simulink model "Impedance_Controller_Week5"  (R2015b)
settings: Solver=ode23t  StartTime=0.0  StopTime=20  MaxStep=1.2  RelTol=1e-5
values from neighbouring files (symbols this model uses):
  B = 0    [ME_495_Position_Control_1.m]    (also in PI_Controller_Week5.m; PI_controller_win1_simulink.m)
  B_desired = testcase(3,i)    [ME_495_Position_Control_1.m]    (also in PI_Controller_Week5.m; PI_controller_win1_simulink.m; TEST.m)
  c = 2*pi*r    (= 0.0552920307032)    [ME_495_Position_Control_1.m]    (also in PI_Controller_Week5.m; PI_controller_win1_simulink.m)
  Fss = testcase(4,i)    [ME_495_Position_Control_1.m]    (also in PI_Controller_Week5.m; PI_controller_win1_simulink.m; TEST.m = 20)
  impulse_duration = input('Duration of the impulse = ')    [ME_495_Position_Control_1.m]    (also in PI_Controller_Week5.m; PI_controller_win1_simulink.m)
  input_mode = input('input mode = ')    [ME_495_Position_Control_1.m]    (also in PI_Controller_Week5.m; PI_controller_win1_simulink.m)
  J = .001    (= 0.001)    [ME_495_Position_Control_1.m]    (also in PI_Controller_Week5.m; PI_controller_win1_simulink.m)
  K_desired = testcase(2,i)    [ME_495_Position_Control_1.m]    (also in PI_Controller_Week5.m; PI_controller_win1_simulink.m; TEST.m)
  Ka = .79    (= 0.79)    [ME_495_Position_Control_1.m]    (also in PI_Controller_Week5.m; PI_controller_win1_simulink.m)
  Ki = wn^2*(r*(M+J*((N^2)/(r^2))))/Ka/Km/N    [PI_Controller_Week5.m]    (also in PI_controller_win1_simulink.m = -f*x*Kp)
  Km = .058    (= 0.058)    [ME_495_Position_Control_1.m]    (also in PI_Controller_Week5.m; PI_controller_win1_simulink.m = 0.11)
  Kp = (wn^2)*r*(M+J/((N*r)^2))/(Ka*Km*N)    [ME_495_Position_Control_1.m]    (also in PI_Controller_Week5.m = (2*zeta*wn*(r*(M+J*((N^2)/(r^2))))-B/r)/(Ka*Km*N); PI_controller_win1_simulink.m = (2*zeta*wn*(r*(M+J/(r^2)))-B/r)/(Ka*Km))
  M = 1    [ME_495_Position_Control_1.m]    (also in PI_Controller_Week5.m; PI_controller_win1_simulink.m; TEST.m)
  M_desired = testcase(1,i)    [ME_495_Position_Control_1.m]    (also in PI_Controller_Week5.m; PI_controller_win1_simulink.m; TEST.m)
  N = 5.9    [ME_495_Position_Control_1.m]    (also in PI_Controller_Week5.m)
  override_flag = 1    [ME_495_Position_Control_1.m]    (also in PI_Controller_Week5.m; PI_controller_win1_simulink.m)
  r = .0176/2    (= 0.0088)    [ME_495_Position_Control_1.m]    (also in PI_Controller_Week5.m; PI_controller_win1_simulink.m)
  Rmot = 3.91    [ME_495_Position_Control_1.m]    (also in PI_Controller_Week5.m = 4; PI_controller_win1_simulink.m = 4)
  target_speed = 5    [ME_495_Position_Control_1.m]    (also in PI_Controller_Week5.m; PI_controller_win1_simulink.m)
  vol_limit = 24    [PI_Controller_Week5.m]
libraries: simulink x3
settings Model: Creator=Jeff  LastModifiedBy=Jeff

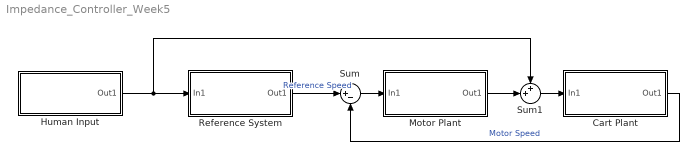
== system Impedance_Controller_Week5 ==
  Cart Plant : Subsystem
  Human Input : Subsystem
  Motor Plant : Subsystem
  Reference System : Subsystem
  Sum : Sum  Inputs=|+-
  Sum1 : Sum  Inputs=++|
  wires:
  Reference System/1(Out1) -> Sum/1  "Reference Speed"
  Cart Plant/1(Out1) -> Sum/2  "Motor Speed"
  Sum1/1 -> Cart Plant/1(In1)
  Sum/1 -> Motor Plant/1(In1)
  Human Input/1(Out1) -> Reference System/1(In1), Sum1/1
  Motor Plant/1(Out1) -> Sum1/2

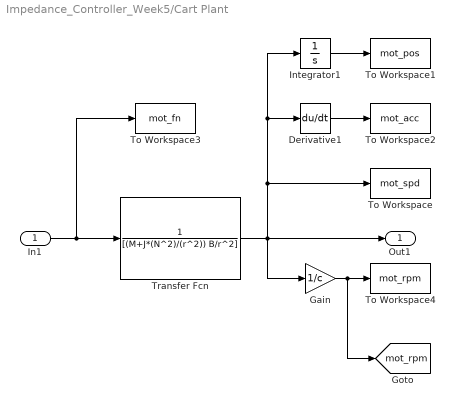
== system Impedance_Controller_Week5/Cart Plant ==
  In1 : Inport
  Derivative1 : Derivative
  Gain : Gain  Gain=1/c
  Integrator1 : Integrator
  To Workspace : ToWorkspace  VariableName=mot_spd  SaveFormat=Timeseries  SampleTime=-1
  To Workspace1 : ToWorkspace  VariableName=mot_pos  SaveFormat=Timeseries  SampleTime=-1
  To Workspace2 : ToWorkspace  VariableName=mot_acc  SaveFormat=Timeseries  SampleTime=-1
  To Workspace3 : ToWorkspace  VariableName=mot_fn  SaveFormat=Timeseries  SampleTime=-1
  To Workspace4 : ToWorkspace  VariableName=mot_rpm  SaveFormat=Timeseries  SampleTime=-1
  Transfer Fcn : TransferFcn  Denominator=[(M+J*(N^2)/(r^2)) B/r^2]
  Out1 : Outport
  tag scope: mot_rpm=global
  wires:
  Integrator1/1 -> To Workspace1/1
  Derivative1/1 -> To Workspace2/1
  In1/1 -> To Workspace3/1, Transfer Fcn/1
  Gain/1 -> [mot_rpm], To Workspace4/1
  Transfer Fcn/1 -> Gain/1, Out1/1, Integrator1/1, Derivative1/1, To Workspace/1

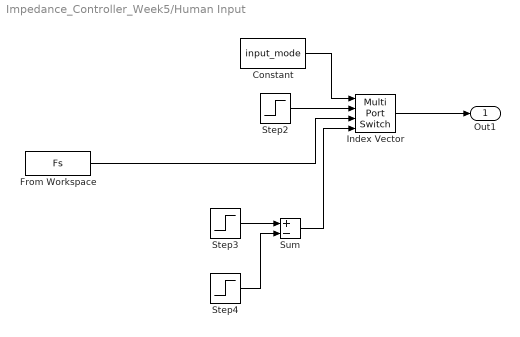
== system Impedance_Controller_Week5/Human Input ==
  Constant : Constant  Value=input_mode
  From Workspace : FromWorkspace  VariableName=Fs  SampleTime=0
  Index Vector : MultiPortSwitch  DataPortOrder=Zero-based contiguous  zeroidx=on
  Step2 : Step  Time=0  After=Fss  SampleTime=0
  Step3 : Step  Time=0  After=Fss  SampleTime=0
  Step4 : Step  Time=impulse_duration  After=Fss  SampleTime=0
  Sum : Sum  Inputs=+-
  Out1 : Outport
  wires:
  From Workspace/1 -> Index Vector/3
  Step2/1 -> Index Vector/2
  Index Vector/1 -> Out1/1
  Constant/1 -> Index Vector/1
  Sum/1 -> Index Vector/4
  Step3/1 -> Sum/1
  Step4/1 -> Sum/2

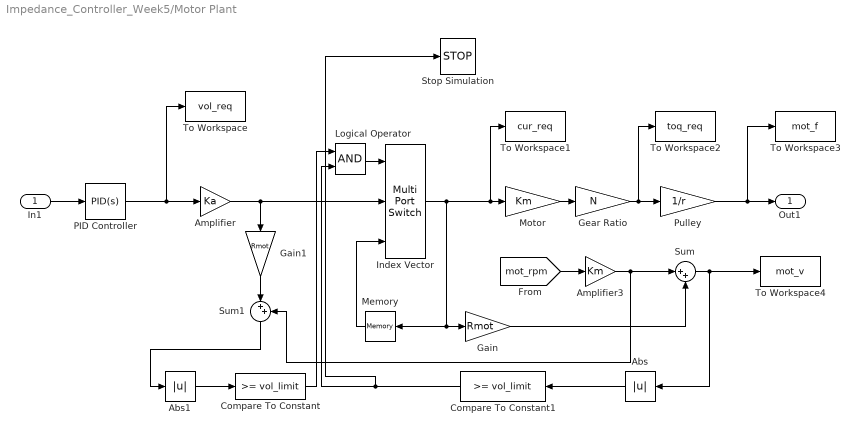
== system Impedance_Controller_Week5/Motor Plant ==
  In1 : Inport
  Abs : Abs
  Abs1 : Abs
  Amplifier : Gain  Gain=Ka
  Amplifier3 : Gain  Gain=Km
  Compare To Constant : simulink/Logic and Bit Operations/Compare To Constant  relop=>=  const=vol_limit  OutDataTypeStr=boolean
  Compare To Constant1 : simulink/Logic and Bit Operations/Compare To Constant  relop=>=  const=vol_limit  OutDataTypeStr=boolean
  Gain : Gain  Gain=Rmot
  Gain1 : Gain  Gain=Rmot
  Gear Ratio : Gain  Gain=N
  Index Vector : MultiPortSwitch  DataPortOrder=Zero-based contiguous  Inputs=2  zeroidx=on
  Logical Operator : Logic  AllPortsSameDT=off  OutDataTypeStr=boolean
  Memory : Memory
  Motor : Gain  Gain=Km
  PID Controller : simulink/Continuous/PID Controller  Controller=PID  TimeDomain=Continuous-time  SampleTime=-1  IntegratorMethod=Forward Euler  FilterMethod=Forward Euler  Form=Parallel  UseFilter=on  ControllerParametersSource=internal  P=Kp  I=Ki  D=0  N=100  InitialConditionSource=internal  InitialConditionForIntegrator=0  InitialConditionForFilter=0  ExternalReset=none  LimitOutput=off  UpperSaturationLimit=inf  LowerSaturationLimit=-inf  LinearizeAsGain=on  AntiWindupMode=none  Kb=1  TrackingMode=off  Kt=1  PParamMin=[]  PParamMax=[]  IParamMin=[]  IParamMax=[]  DParamMin=[]  DParamMax=[]  NParamMin=[]  NParamMax=[]  KbParamMin=[]  KbParamMax=[]  KtParamMin=[]  KtParamMax=[]  POutMin=[]  POutMax=[]  IOutMin=[]  IOutMax=[]  DOutMin=[]  DOutMax=[]  NOutMin=[]  NOutMax=[]  KbOutMin=[]  KbOutMax=[]  KtOutMin=[]  KtOutMax=[]  IntegratorOutMin=[]  IntegratorOutMax=[]  FilterOutMin=[]  FilterOutMax=[]  SumOutMin=[]  SumOutMax=[]  SumI1OutMin=[]  SumI1OutMax=[]  SumI2OutMin=[]  SumI2OutMax=[]  SumI3OutMin=[]  SumI3OutMax=[]  SumDOutMin=[]  SumDOutMax=[]  SaturationOutMin=[]  SaturationOutMax=[]  IntegratorContinuousStateAttributes=''  IntegratorStateMustResolveToSignalObject=off  IntegratorRTWStateStorageClass=Auto  FilterContinuousStateAttributes=''  FilterStateMustResolveToSignalObject=off  FilterRTWStateStorageClass=Auto  DifferentiatorICPrevScaledInput=0  DifferentiatorOutMin=[]  DifferentiatorOutMax=[]
  Pulley : Gain  Gain=1/r
  Stop Simulation : Stop
  Sum : Sum  Inputs=|++
  Sum1 : Sum  Inputs=|++
  To Workspace : ToWorkspace  VariableName=vol_req  SaveFormat=Timeseries  SampleTime=-1
  To Workspace1 : ToWorkspace  VariableName=cur_req  SaveFormat=Timeseries  SampleTime=-1
  To Workspace2 : ToWorkspace  VariableName=toq_req  SaveFormat=Timeseries  SampleTime=-1
  To Workspace3 : ToWorkspace  VariableName=mot_f  SaveFormat=Timeseries  SampleTime=-1
  To Workspace4 : ToWorkspace  VariableName=mot_v  SaveFormat=Timeseries  SampleTime=-1
  Out1 : Outport
  wires:
  In1/1 -> PID Controller/1
  Index Vector/1 -> Memory/1, Gain/1, To Workspace1/1, Motor/1
  Pulley/1 -> To Workspace3/1, Out1/1
  Gain/1 -> Sum/2
  Amplifier3/1 -> Sum/1, Sum1/2
  Sum/1 -> Abs/1, To Workspace4/1
  [mot_rpm] -> Amplifier3/1
  Motor/1 -> Gear Ratio/1
  Gear Ratio/1 -> To Workspace2/1, Pulley/1
  PID Controller/1 -> To Workspace/1, Amplifier/1
  Amplifier/1 -> Gain1/1, Index Vector/2
  Memory/1 -> Index Vector/3
  Gain1/1 -> Sum1/1
  Sum1/1 -> Abs1/1
  Compare To Constant/1 -> Logical Operator/1
  Logical Operator/1 -> Index Vector/1
  Abs/1 -> Compare To Constant1/1
  Abs1/1 -> Compare To Constant/1
  Compare To Constant1/1 -> Stop Simulation/1, Logical Operator/2

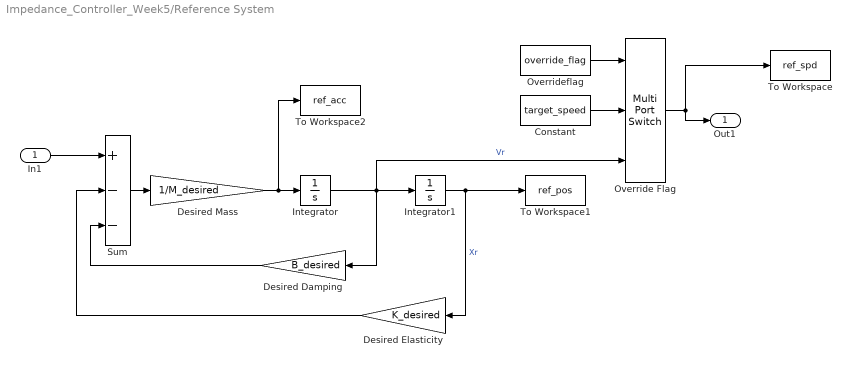
== system Impedance_Controller_Week5/Reference System ==
  In1 : Inport
  Constant : Constant  Value=target_speed
  Desired Damping : Gain  Gain=B_desired
  Desired Elasticity : Gain  Gain=K_desired
  Desired Mass : Gain  Gain=1/M_desired
  Integrator : Integrator
  Integrator1 : Integrator
  Override Flag : MultiPortSwitch  DataPortOrder=Zero-based contiguous  Inputs=2  zeroidx=on
  Overrideflag : Constant  Value=override_flag
  Sum : Sum  Inputs=+--
  To Workspace : ToWorkspace  VariableName=ref_spd  SaveFormat=Timeseries  SampleTime=-1
  To Workspace1 : ToWorkspace  VariableName=ref_pos  SaveFormat=Timeseries  SampleTime=-1
  To Workspace2 : ToWorkspace  VariableName=ref_acc  SaveFormat=Timeseries  SampleTime=-1
  Out1 : Outport
  wires:
  In1/1 -> Sum/1
  Sum/1 -> Desired Mass/1
  Integrator/1 -> Override Flag/3, Desired Damping/1, Integrator1/1  "Vr"
  Desired Mass/1 -> To Workspace2/1, Integrator/1
  Desired Damping/1 -> Sum/3
  Integrator1/1 -> Desired Elasticity/1, To Workspace1/1  "Xr"
  Desired Elasticity/1 -> Sum/2
  Override Flag/1 -> Out1/1, To Workspace/1
  Overrideflag/1 -> Override Flag/1
  Constant/1 -> Override Flag/2
